simulink model "Der_Faux_FPGA_V2"  (R2020a)
settings: Solver=FixedStepDiscrete  StartTime=0.0  StopTime=0.84375  FixedStep=1/fs_sim  RelTol=1e-3
values from neighbouring files (symbols this model uses):
  ADC_res = 5    [Der_Faux_ctr_FPGA.m]
  ADC_res_G4 = 8    [Der_Faux_ctr_FPGA.m]
  C10 = 680e-12    (= 6.8e-10)    [Der_Faux_ctr_FPGA.m]
  C11 = 1e-9    (= 1e-09)    [Der_Faux_ctr_FPGA.m]
  C12 = 68e-9    (= 6.8e-08)    [Der_Faux_ctr_FPGA.m]
  C13 = 150e-9    (= 1.5e-07)    [Der_Faux_ctr_FPGA.m]
  C17 = 1e-6    (= 1e-06)    [Der_Faux_ctr_FPGA.m]
  C18 = 100e-9    (= 1e-07)    [Der_Faux_ctr_FPGA.m]
  C20 = 1e-6    (= 1e-06)    [Der_Faux_ctr_FPGA.m]
  C5 = 100e-12    (= 1e-10)    [Der_Faux_ctr_FPGA.m]
  C7 = 1e-6    (= 1e-06)    [Der_Faux_ctr_FPGA.m]
  D4_FL = D4_opt.FractionLength    [Der_Faux_ctr_FPGA.m]
  D4_opt = sfi(D4,len_D)    [Der_Faux_ctr_FPGA.m]
  D4_WL = D4_opt.WordLength    [Der_Faux_ctr_FPGA.m]
  D7_FL = D7_opt.FractionLength    [Der_Faux_ctr_FPGA.m]
  D7_opt = sfi(D7,len_D)    [Der_Faux_ctr_FPGA.m]
  D7_WL = D7_opt.WordLength    [Der_Faux_ctr_FPGA.m]
  D8_FL = D8_opt.FractionLength    [Der_Faux_ctr_FPGA.m]
  D8_opt = sfi(D8,len_D)    [Der_Faux_ctr_FPGA.m]
  D8_WL = D8_opt.WordLength    [Der_Faux_ctr_FPGA.m]
  Dcs1_FL = Dcs1_opt.FractionLength    [Der_Faux_ctr_FPGA.m]
  Dcs1_opt = sfi(Dcs1,len_D)    [Der_Faux_ctr_FPGA.m]
  Dcs1_WL = Dcs1_opt.WordLength    [Der_Faux_ctr_FPGA.m]
  Dcs2_FL = Dcs2_opt.FractionLength    [Der_Faux_ctr_FPGA.m]
  Dcs2_WL = Dcs2_opt.WordLength    [Der_Faux_ctr_FPGA.m]
  FP_frac = FP_len-10    (= 36)    [Der_Faux_ctr_FPGA.m]
  FP_len = 46    [Der_Faux_ctr_FPGA.m]
  fs = 48000    [Der_Faux_ctr_FPGA.m]
  fs_sim = fs*ovs    (= 6144000)    [Der_Faux_ctr_FPGA.m]
  G0 = 1/4.7e3    (= 0.000212765957447)    [Der_Faux_ctr_FPGA.m]
  G1 = 1/4.7e3    (= 0.000212765957447)    [Der_Faux_ctr_FPGA.m]
  G10 = 1/12e3    (= 8.33333333333e-05)    [Der_Faux_ctr_FPGA.m]
  G11 = 1/12e3    (= 8.33333333333e-05)    [Der_Faux_ctr_FPGA.m]
  G12 = 1/12e3    (= 8.33333333333e-05)    [Der_Faux_ctr_FPGA.m]
  G13 = 1/47e3    (= 2.12765957447e-05)    [Der_Faux_ctr_FPGA.m]
  G14 = 1/22e3    (= 4.54545454545e-05)    [Der_Faux_ctr_FPGA.m]
  G15 = 1/12e3    (= 8.33333333333e-05)    [Der_Faux_ctr_FPGA.m]
  G16 = 1/12e3    (= 8.33333333333e-05)    [Der_Faux_ctr_FPGA.m]
  G17 = 1/12e3    (= 8.33333333333e-05)    [Der_Faux_ctr_FPGA.m]
  G18 = 1/2.7e3    (= 0.00037037037037)    [Der_Faux_ctr_FPGA.m]
  G19 = 1/20e3    (= 5e-05)    [Der_Faux_ctr_FPGA.m]
  G20 = 1/10e3    (= 0.0001)    [Der_Faux_ctr_FPGA.m]
  G21 = 1/10e3    (= 0.0001)    [Der_Faux_ctr_FPGA.m]
  G5 = 1/22e3    (= 4.54545454545e-05)    [Der_Faux_ctr_FPGA.m]
  G7 = 1/12e3    (= 8.33333333333e-05)    [Der_Faux_ctr_FPGA.m]
  Gdem = 0.00096    [Der_Faux_ctr_FPGA.m]
  Gmod = 0.00096    [Der_Faux_ctr_FPGA.m]
  Gvar1_N = fi(Gvar1_N,0,ADC_res,0)    [Der_Faux_ctr_FPGA.m]
  Gvar2_N = fi(Gvar2_N,0,ADC_res,0)    [Der_Faux_ctr_FPGA.m]
  Gvar3_N = fi(Gvar3_N,0,ADC_res,0)    [Der_Faux_ctr_FPGA.m]
  Gvar4_N = fi(Gvar4_N,0,ADC_res_G4,0)    [Der_Faux_ctr_FPGA.m]
  input_space = linspace(0,2^ADC_res-1,2^ADC_res)    [Der_Faux_ctr_FPGA.m]
  input_space_G4 = linspace(0,2^ADC_res_G4-1,2^ADC_res_G4)    [Der_Faux_ctr_FPGA.m]
  input_spcae_extended = linspace(0,(2^ADC_res)^3-1,(2^ADC_res)^3)    [Der_Faux_ctr_FPGA.m]
  limit_Faux = 4.5    [Der_Faux_ctr_FPGA.m]
  limit_PT2399 = 2.5    [Der_Faux_ctr_FPGA.m]
  LUT_cd = fi(LUT_cd,0,LUT_cd_res,0)    [Der_Faux_ctr_FPGA.m]
  LUT_Gvar1_opt = sfi(LUT_Gvar1, len1)    [Der_Faux_ctr_FPGA.m]
  LUT_Gvar2_reversed_opt = sfi(LUT_Gvar2_reversed, len2)    [Der_Faux_ctr_FPGA.m]
  LUT_Gvar3_opt = sfi(LUT_Gvar3, len3)    [Der_Faux_ctr_FPGA.m]
  LUT_Z22a_opt = sfi(LUT_Z22a, len_LUT22a)    [Der_Faux_ctr_FPGA.m]
  LUT_Z22b_opt = sfi(LUT_Z22b, len_LUT22b)    [Der_Faux_ctr_FPGA.m]
  LUT_Z23a_opt = sfi(LUT_Z23a, len_Z23a)    [Der_Faux_ctr_FPGA.m]
  LUT_Z23b_opt = sfi(LUT_Z23b, len_Z23b)    [Der_Faux_ctr_FPGA.m]
  LUT_Z24a_opt = sfi(LUT_Z24a, len_LUT24a)    [Der_Faux_ctr_FPGA.m]
  LUT_Z24b_opt = sfi(LUT_Z24b, len_LUT24b)    [Der_Faux_ctr_FPGA.m]
  LUT_Z25a_opt = sfi(LUT_Z25a, len_LUT25a)    [Der_Faux_ctr_FPGA.m]
  LUT_Z25b_opt = sfi(LUT_Z25b, len_LUT25b)    [Der_Faux_ctr_FPGA.m]
  N4_FL = N4_opt.FractionLength    [Der_Faux_ctr_FPGA.m]
  N4_opt = sfi(N4,len_N)    [Der_Faux_ctr_FPGA.m]
  N4_WL = N4_opt.WordLength    [Der_Faux_ctr_FPGA.m]
  N7_FL = N7_opt.FractionLength    [Der_Faux_ctr_FPGA.m]
  N7_opt = sfi(N7,len_N)    [Der_Faux_ctr_FPGA.m]
  N7_WL = N7_opt.WordLength    [Der_Faux_ctr_FPGA.m]
  N8_FL = N8_opt.FractionLength    [Der_Faux_ctr_FPGA.m]
  N8_opt = sfi(N8,len_N)    [Der_Faux_ctr_FPGA.m]
  N8_WL = N8_opt.WordLength    [Der_Faux_ctr_FPGA.m]
  Ncs1_FL = Ncs1_opt.FractionLength    [Der_Faux_ctr_FPGA.m]
  Ncs1_opt = sfi(Ncs1,len_N)    [Der_Faux_ctr_FPGA.m]
  Ncs1_WL = Ncs1_opt.WordLength    [Der_Faux_ctr_FPGA.m]
  Ncs2_FL = Ncs2_opt.FractionLength    [Der_Faux_ctr_FPGA.m]
  Ncs2_WL = Ncs2_opt.WordLength    [Der_Faux_ctr_FPGA.m]
  shift_reg_size = 8*44000    (= 352000)    [Der_Faux_ctr_FPGA.m]
  use_stimuli = [true,true,true,true]    [Der_Faux_ctr_FPGA.m]
  w1 = 1e6    (= 1000000)    [Der_Faux_ctr_FPGA.m]
  w3 = 1e6    (= 1000000)    [Der_Faux_ctr_FPGA.m]
  w4 = 1e6    (= 1000000)    [Der_Faux_ctr_FPGA.m]
  w5 = 1e6    (= 1000000)    [Der_Faux_ctr_FPGA.m]
  w8 = 2*pi*3e6    (= 18849555.9215)    [Der_Faux_ctr_FPGA.m]
  WL_RAM = 5    [Der_Faux_ctr_FPGA.m]
undefined symbols (not defined in the file or in its folder): D10_FL, D10_opt, D10_WL, D11_FL, D11_opt, D11_WL, D13_FL, D13_opt, D13_WL, D16_FL, D16_opt, D16_WL, D20_FL, D20_opt, D20_WL, D21_FL, D21_opt, D21_WL, D26_FL, D26_opt, D26_WL, D27_FL, D27_opt, D27_WL, D28_FL, D28_opt, D28_WL, D29_FL, D29_opt, D29_WL, D30_FL, D30_opt, D30_WL, Dcs2, DiscIntNeverNeededParam, N10_FL, N10_opt, N10_WL, N11_FL, N11_opt, N11_WL, N13_FL, N13_opt, N13_WL, N16_FL, N16_opt, N16_WL, N20_FL, N20_opt, N20_WL, N21_FL, N21_opt, N21_WL, N26_FL, N26_opt, N26_WL, N27_FL, N27_opt, N27_WL, N28_FL ... (+13)
libraries: simulink x18, hdlsllib x4
(part 1 of 2)
settings Model: Creator=Donut  LastModifiedBy=Donut
settings OptimizationCC: BlockReduction=off  ConditionallyExecuteInputs=off  DefaultParameterBehavior=Inlined
settings DebuggingCC: SignalRangeChecking=warning  AlgebraicLoopMsg=error  SingleTaskRateTransMsg=error  ParameterOverflowMsg=warning  ParameterUnderflowMsg=warning  UnnecessaryDatatypeConvMsg=warning
settings HardwareCC: ProdBitPerPointer=32  ProdBitPerSizeT=32  ProdBitPerPtrDiffT=32  ProdLargestAtomicFloat=None  ProdIntDivRoundTo=Undefined  ProdEndianess=Unspecified  ProdWordSize=32  ProdHWDeviceType=ASIC/FPGA->ASIC/FPGA  TargetBitPerPointer=64  TargetBitPerSizeT=64  TargetBitPerPtrDiffT=64  TargetLongLongMode=on  TargetIntDivRoundTo=Zero  TargetEndianess=LittleEndian  TargetWordSize=64  TargetHWDeviceType=Custom Processor->MATLAB Host Computer  ProdEqTarget=off
settings SFSimCC: CustomCodeUndefinedFunction=UseInterfaceOnly

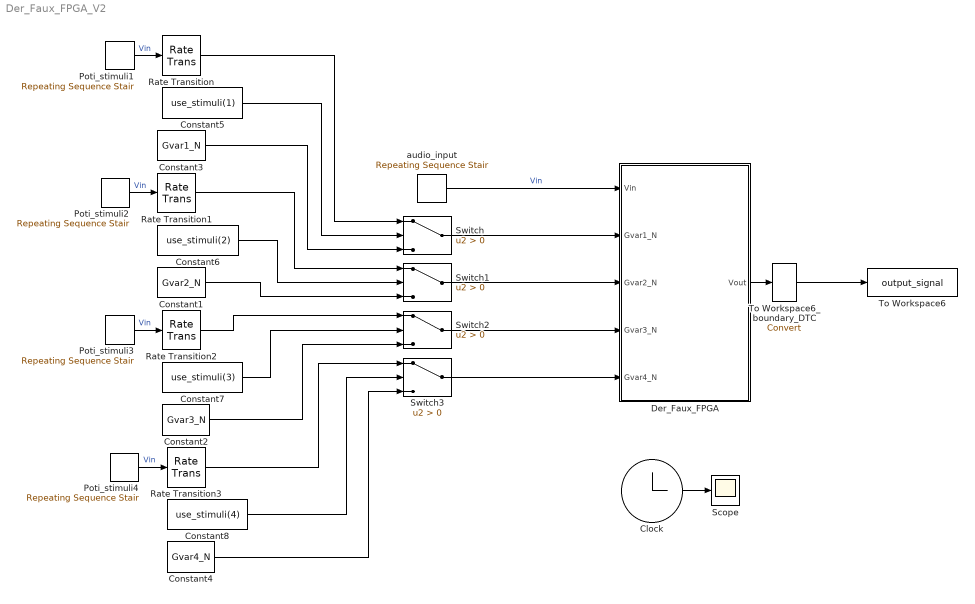
== system Der_Faux_FPGA_V2 ==
  Clock : Clock
  Constant1 : Constant  Value=Gvar2_N  OutDataTypeStr=fixdt(0,ADC_res,0)  SampleTime=1/fs_sim  LockScale=on
  Constant2 : Constant  Value=Gvar3_N  OutDataTypeStr=fixdt(0,ADC_res,0)  SampleTime=1/fs_sim  LockScale=on
  Constant3 : Constant  Value=Gvar1_N  OutDataTypeStr=fixdt(0,ADC_res,0)  SampleTime=1/fs_sim  LockScale=on
  Constant4 : Constant  Value=Gvar4_N  OutDataTypeStr=fixdt(0,ADC_res_G4,0)  SampleTime=1/(fs_sim)  LockScale=on
  Constant5 : Constant  Value=use_stimuli(1)  OutDataTypeStr=boolean  SampleTime=1/fs_sim  LockScale=on
  Constant6 : Constant  Value=use_stimuli(2)  OutDataTypeStr=boolean  SampleTime=1/fs_sim  LockScale=on
  Constant7 : Constant  Value=use_stimuli(3)  OutDataTypeStr=boolean  SampleTime=1/fs_sim  LockScale=on
  Constant8 : Constant  Value=use_stimuli(4)  OutDataTypeStr=boolean  SampleTime=1/(fs_sim)  LockScale=on
  Der_Faux_FPGA : Subsystem
  "Poti_stimuli1 " : simulink/Sources/Repeating Sequence Stair  OutValues=poti_stimuli1'  tsamp=1/fs  OutMin=[]  OutMax=[]  OutDataTypeStr=fixdt(0,ADC_res,0)  OutputDataTypeScalingMode=Specify via dialog  OutDataType=fixdt(0,ADC_res,0)  ConRadixGroup=Best Precision: Vector-wise  OutScaling=[]
      settings: LockScale=on
  "Poti_stimuli2 " : simulink/Sources/Repeating Sequence Stair  OutValues=poti_stimuli2'  tsamp=1/fs  OutMin=[]  OutMax=[]  OutDataTypeStr=fixdt(0,ADC_res,0)  OutputDataTypeScalingMode=Specify via dialog  OutDataType=fixdt(0,ADC_res,0)  ConRadixGroup=Best Precision: Vector-wise  OutScaling=[]
      settings: LockScale=on
  Poti_stimuli3 : simulink/Sources/Repeating Sequence Stair  OutValues=poti_stimuli3'  tsamp=1/fs  OutMin=[]  OutMax=[]  OutDataTypeStr=fixdt(0,ADC_res,0)  OutputDataTypeScalingMode=Specify via dialog  OutDataType=fixdt(0,ADC_res,0)  ConRadixGroup=Best Precision: Vector-wise  OutScaling=[]
      settings: LockScale=on
  Poti_stimuli4 : simulink/Sources/Repeating Sequence Stair  OutValues=poti_stimuli4'  tsamp=1/fs  OutMin=[]  OutMax=[]  OutDataTypeStr=fixdt(0,ADC_res_G4,0)  OutputDataTypeScalingMode=Specify via dialog  OutDataType=fixdt(0,ADC_res_G4,0)  ConRadixGroup=Best Precision: Vector-wise  OutScaling=[]
      settings: LockScale=on
  Rate Transition{,1..3} (4 alike) : RateTransition  OutPortSampleTime=1/fs_sim
  Scope : Scope
  Switch : Switch  Criteria=u2 > Threshold  OutDataTypeStr=fixdt(0,ADC_res,0)
      settings: LockScale=on
  Switch1 : Switch  Criteria=u2 > Threshold  OutDataTypeStr=fixdt(0,ADC_res,0)
      settings: LockScale=on
  Switch2 : Switch  Criteria=u2 > Threshold  OutDataTypeStr=fixdt(0,ADC_res,0)
      settings: LockScale=on
  Switch3 : Switch  Criteria=u2 > Threshold  OutDataTypeStr=fixdt(0,ADC_res_G4,0)
      settings: LockScale=on
  To Workspace6 : ToWorkspace  VariableName=output_signal  SaveFormat=Timeseries  SampleTime=1/fs
  To Workspace6_boundary_DTC : DataTypeConversion  SaturateOnIntegerOverflow=on  RndMeth=Zero
  audio_input : simulink/Sources/Repeating Sequence Stair  OutValues=audio'  tsamp=1/fs  OutMin=[]  OutMax=[]  OutDataTypeStr=fixdt(1,16,15)  OutputDataTypeScalingMode=Specify via dialog  OutDataType=fixdt(1,16,15)  ConRadixGroup=Best Precision: Vector-wise  OutScaling=[]
      settings: LockScale=on
  wires:
  Clock/1 -> Scope/1
  Constant5/1 -> Switch/2
  Constant6/1 -> Switch1/2
  Constant8/1 -> Switch3/2
  Constant7/1 -> Switch2/2
  Constant3/1 -> Switch/3
  Constant1/1 -> Switch1/3
  Constant2/1 -> Switch2/3
  Constant4/1 -> Switch3/3
  "Poti_stimuli1 "/1 -> Rate Transition/1  "Vin"
  Rate Transition/1 -> Switch/1
  Rate Transition3/1 -> Switch3/1
  "Poti_stimuli2 "/1 -> Rate Transition1/1  "Vin"
  Poti_stimuli3/1 -> Rate Transition2/1  "Vin"
  Poti_stimuli4/1 -> Rate Transition3/1  "Vin"
  Rate Transition1/1 -> Switch1/1
  Rate Transition2/1 -> Switch2/1
  Switch/1 -> Der_Faux_FPGA/2(Gvar1_N)
  Switch1/1 -> Der_Faux_FPGA/3(Gvar2_N)
  Switch3/1 -> Der_Faux_FPGA/5(Gvar4_N)
  audio_input/1 -> Der_Faux_FPGA/1(Vin)  "Vin"
  Switch2/1 -> Der_Faux_FPGA/4(Gvar3_N)
  Der_Faux_FPGA/1(Vout) -> To Workspace6_boundary_DTC/1
  To Workspace6_boundary_DTC/1 -> To Workspace6/1

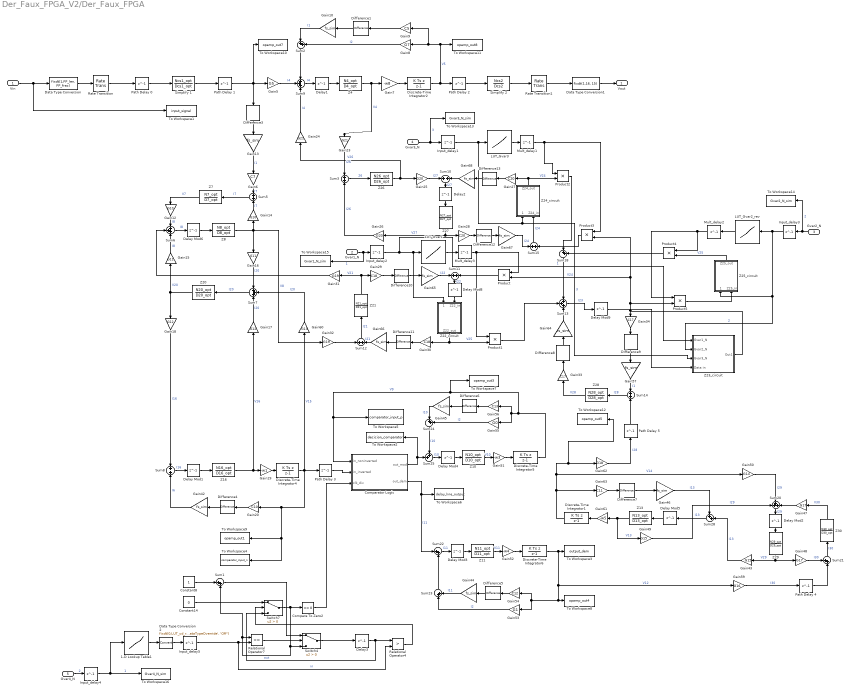
== system Der_Faux_FPGA_V2/Der_Faux_FPGA ==
  Vin : Inport  OutDataTypeStr=fixdt(1,16, 15)  SampleTime=1/fs  LockScale=on
  Gvar1_N : Inport  Port=2  OutDataTypeStr=fixdt(0,ADC_res,0, 'DataTypeOverride', 'Off')  SampleTime=1/fs_sim  LockScale=on
  Gvar2_N : Inport  Port=3  OutDataTypeStr=fixdt(0,ADC_res,0, 'DataTypeOverride', 'Off')  SampleTime=1/fs_sim  LockScale=on
  Gvar3_N : Inport  Port=4  OutDataTypeStr=fixdt(0,ADC_res,0, 'DataTypeOverride', 'Off')  SampleTime=1/fs_sim  LockScale=on
  Gvar4_N : Inport  Port=5  OutDataTypeStr=fixdt(0,ADC_res_G4,0, 'DataTypeOverride', 'Off')  SampleTime=1/(fs_sim)  LockScale=on
  1-D Lookup Table1 : Lookup_n-D  NumberOfTableDimensions=1  LookupTableObject=''  BreakpointsForDimension1=input_space_G4  BreakpointsForDimension1FirstPoint=10  BreakpointsForDimension2FirstPoint=10  BreakpointsForDimension1Spacing=12  BreakpointsForDimension2Spacing=12  BreakpointsForDimension1DataTypeStr=Inherit: Inherit from 'Breakpoint data'  IndexSearchMethod=Evenly spaced points  Table=LUT_cd  TableDataTypeStr=Inherit: Inherit from 'Table data'  InterpMethod=Flat  DiagnosticForOutOfRangeInput=Error  InternalRulePriority=Speed  OutDataTypeStr=Inherit: Inherit from 'Table data'  RndMeth=Simplest  InputSameDT=on  LockScale=on
  Comparator Logic : Subsystem
  Compare To Zero2 : simulink/Logic and Bit Operations/Compare To Zero  relop===  OutDataTypeStr=boolean
  Constant14 : Constant  Value=0  OutDataTypeStr=fixdt(0,LUT_cd_res,0, 'DataTypeOverride', 'Off')  SampleTime=1/(fs_sim)  LockScale=on
  Constant8 : Constant  OutDataTypeStr=fixdt(0,LUT_cd_res,0, 'DataTypeOverride', 'Off')  SampleTime=1/(fs_sim)  LockScale=on
  Data Type Conversion : DataTypeConversion  OutDataTypeStr=fixdt(1,FP_len, FP_frac)  SaturateOnIntegerOverflow=on
  Data Type Conversion1 : DataTypeConversion  OutDataTypeStr=fixdt(1,16, 15)  SaturateOnIntegerOverflow=on  LockScale=on
  Data Type Conversion2 : DataTypeConversion  OutDataTypeStr=fixdt(0,LUT_cd_res,0, 'DataTypeOverride', 'Off')  LockScale=on
  Delay Mod{1..6,8..9} (8 alike) : Delay  DelayLength=1  InitialCondition=0  SampleTime=1/fs_sim
  Delay1 : Delay  DelayLength=1
  Delay2 : Delay  DelayLength=1
  Delay3 : Delay  DelayLength=1  SampleTime=1/(fs_sim)
  Difference{1,3..13} (12 alike) : simulink/Discrete/Difference  ICPrevInput=0.0  OutMin=[]  OutMax=[]  OutDataTypeStr=fixdt(1,FP_len, FP_frac)  OutputDataTypeScalingMode=Specify via dialog  OutDataType=fixdt(1,FP_len, FP_frac)  OutScaling=[]  DoSatur=on
  Discrete-Time Integrator{1,4..6} (4 alike) : DiscreteIntegrator  IntegratorMethod=Integration: Backward Euler  SampleTime=1/fs_sim  OutDataTypeStr=fixdt(1,FP_len, FP_frac)  SaturateOnIntegerOverflow=on  LimitOutput=on  UpperSaturationLimit=limit_PT2399  LowerSaturationLimit=-limit_PT2399  ICPrevOutput=DiscIntNeverNeededParam  ICPrevScaledInput=DiscIntNeverNeededParam
  Discrete-Time Integrator2 : DiscreteIntegrator  IntegratorMethod=Integration: Backward Euler  SampleTime=1/fs_sim  OutDataTypeStr=fixdt(1,FP_len, FP_frac)  SaturateOnIntegerOverflow=on  LimitOutput=on  UpperSaturationLimit=limit_Faux  LowerSaturationLimit=-limit_Faux  ICPrevOutput=DiscIntNeverNeededParam  ICPrevScaledInput=DiscIntNeverNeededParam
  Gain{10,13,42,44..46,57,64..68} (12 alike) : Gain  Gain=fs_sim  OutDataTypeStr=fixdt(1,FP_len, FP_frac)  SaturateOnIntegerOverflow=on
  Gain12 : Gain  Gain=G10  OutDataTypeStr=fixdt(1,FP_len, FP_frac)  SaturateOnIntegerOverflow=on
  Gain14 : Gain  Gain=G10  OutDataTypeStr=fixdt(1,FP_len, FP_frac)  SaturateOnIntegerOverflow=on
  Gain15 : Gain  Gain=G11  OutDataTypeStr=fixdt(1,FP_len, FP_frac)  SaturateOnIntegerOverflow=on
  Gain16 : Gain  Gain=G11  OutDataTypeStr=fixdt(1,FP_len, FP_frac)  SaturateOnIntegerOverflow=on
  Gain17 : Gain  Gain=G12  OutDataTypeStr=fixdt(1,FP_len, FP_frac)  SaturateOnIntegerOverflow=on
  Gain18 : Gain  Gain=G12  OutDataTypeStr=fixdt(1,FP_len, FP_frac)  SaturateOnIntegerOverflow=on
  Gain19 : Gain  Gain=-w1  OutDataTypeStr=fixdt(1,FP_len, FP_frac)  SaturateOnIntegerOverflow=on
  Gain20 : Gain  Gain=C10  OutDataTypeStr=fixdt(1,FP_len, FP_frac)  SaturateOnIntegerOverflow=on
  Gain23 : Gain  Gain=G21  OutDataTypeStr=fixdt(1,FP_len, FP_frac)  SaturateOnIntegerOverflow=on
  Gain24 : Gain  Gain=G21  OutDataTypeStr=fixdt(1,FP_len, FP_frac)  SaturateOnIntegerOverflow=on
  Gain25 : Gain  Gain=G20  OutDataTypeStr=fixdt(1,FP_len, FP_frac)  SaturateOnIntegerOverflow=on
  Gain26 : Gain  Gain=G20  OutDataTypeStr=fixdt(1,FP_len, FP_frac)  SaturateOnIntegerOverflow=on
  Gain27 : Gain  Gain=C20  OutDataTypeStr=fixdt(1,FP_len, FP_frac)  SaturateOnIntegerOverflow=on
  Gain28 : Gain  Gain=C20  OutDataTypeStr=fixdt(1,FP_len, FP_frac)  SaturateOnIntegerOverflow=on
  Gain29 : Gain  Gain=C18  OutDataTypeStr=fixdt(1,FP_len, FP_frac)  SaturateOnIntegerOverflow=on
  Gain30 : Gain  Gain=C18  OutDataTypeStr=fixdt(1,FP_len, FP_frac)  SaturateOnIntegerOverflow=on
  Gain31 : Gain  Gain=G19  OutDataTypeStr=fixdt(1,FP_len, FP_frac)  SaturateOnIntegerOverflow=on
  Gain32 : Gain  Gain=G19  OutDataTypeStr=fixdt(1,FP_len, FP_frac)  SaturateOnIntegerOverflow=on
  Gain33 : Gain  Gain=C17  OutDataTypeStr=fixdt(1,FP_len, FP_frac)  SaturateOnIntegerOverflow=on
  Gain34 : Gain  Gain=C17  OutDataTypeStr=fixdt(1,FP_len, FP_frac)  SaturateOnIntegerOverflow=on
  Gain43 : Gain  Gain=G15  OutDataTypeStr=fixdt(1,FP_len, FP_frac)  SaturateOnIntegerOverflow=on
  Gain47 : Gain  Gain=G17  OutDataTypeStr=fixdt(1,FP_len, FP_frac)  SaturateOnIntegerOverflow=on
  Gain48 : Gain  Gain=G17  OutDataTypeStr=fixdt(1,FP_len, FP_frac)  SaturateOnIntegerOverflow=on
  Gain49 : Gain  Gain=G15  OutDataTypeStr=fixdt(1,FP_len, FP_frac)  SaturateOnIntegerOverflow=on
  Gain5 : Gain  Gain=G5  OutDataTypeStr=fixdt(1,FP_len, FP_frac)  SaturateOnIntegerOverflow=on
  Gain50 : Gain  Gain=G14  OutDataTypeStr=fixdt(1,FP_len, FP_frac)  SaturateOnIntegerOverflow=on
  Gain51 : Gain  Gain=-w3  OutDataTypeStr=fixdt(1,FP_len, FP_frac)  SaturateOnIntegerOverflow=on
  Gain52 : Gain  Gain=-w4  OutDataTypeStr=fixdt(1,FP_len, FP_frac)  SaturateOnIntegerOverflow=on
  Gain53 : Gain  Gain=G1  OutDataTypeStr=fixdt(1,FP_len, FP_frac)  SaturateOnIntegerOverflow=on
  Gain54 : Gain  Gain=C12  OutDataTypeStr=fixdt(1,FP_len, FP_frac)  SaturateOnIntegerOverflow=on
  Gain55 : Gain  Gain=G0  OutDataTypeStr=fixdt(1,FP_len, FP_frac)  SaturateOnIntegerOverflow=on
  Gain56 : Gain  Gain=C13  OutDataTypeStr=fixdt(1,FP_len, FP_frac)  SaturateOnIntegerOverflow=on
  Gain59 : Gain  Gain=G16  OutDataTypeStr=fixdt(1,FP_len, FP_frac)  SaturateOnIntegerOverflow=on
  Gain6 : Gain  Gain=C7  OutDataTypeStr=fixdt(1,FP_len, FP_frac)  SaturateOnIntegerOverflow=on
  Gain60 : Gain  Gain=G13  OutDataTypeStr=fixdt(1,FP_len, FP_frac)  SaturateOnIntegerOverflow=on
  Gain61 : Gain  Gain=-w5  OutDataTypeStr=fixdt(1,FP_len, FP_frac)  SaturateOnIntegerOverflow=on
  Gain62 : Gain  Gain=G18  OutDataTypeStr=fixdt(1,FP_len, FP_frac)  SaturateOnIntegerOverflow=on
  Gain63 : Gain  Gain=C11  OutDataTypeStr=fixdt(1,FP_len, FP_frac)  SaturateOnIntegerOverflow=on
  Gain7 : Gain  Gain=-w8  OutDataTypeStr=fixdt(1,FP_len, FP_frac)  SaturateOnIntegerOverflow=on
  Gain8 : Gain  Gain=G7  OutDataTypeStr=fixdt(1,FP_len, FP_frac)  SaturateOnIntegerOverflow=on
  Gain9 : Gain  Gain=C5  OutDataTypeStr=fixdt(1,FP_len, FP_frac)  SaturateOnIntegerOverflow=on
  Input_delay{1..4} (4 alike) : Delay  DelayLength=1
  Input_delay5 : Delay  DelayLength=1  InitialCondition=1  SampleTime=1/(fs_sim)
  "LUT_Gvar1 " : Lookup_n-D  NumberOfTableDimensions=1  LookupTableObject=''  BreakpointsForDimension1=input_space  BreakpointsForDimension1FirstPoint=10  BreakpointsForDimension2FirstPoint=10  BreakpointsForDimension1Spacing=12  BreakpointsForDimension2Spacing=12  IndexSearchMethod=Evenly spaced points  Table=LUT_Gvar1_opt  TableDataTypeStr=Inherit: Inherit from 'Table data'  InterpMethod=Flat  DiagnosticForOutOfRangeInput=Error  InternalRulePriority=Speed  OutDataTypeStr=Inherit: Inherit from 'Table data'  RndMeth=Simplest  InputSameDT=on  LockScale=on
  LUT_Gvar2_rev : Lookup_n-D  NumberOfTableDimensions=1  LookupTableObject=''  BreakpointsForDimension1=input_space  BreakpointsForDimension1FirstPoint=10  BreakpointsForDimension2FirstPoint=10  BreakpointsForDimension1Spacing=12  BreakpointsForDimension2Spacing=12  BreakpointsForDimension1DataTypeStr=Inherit: Inherit from 'Breakpoint data'  IndexSearchMethod=Evenly spaced points  Table=LUT_Gvar2_reversed_opt  TableDataTypeStr=Inherit: Inherit from 'Table data'  InterpMethod=Flat  DiagnosticForOutOfRangeInput=Error  InternalRulePriority=Speed  OutDataTypeStr=Inherit: Inherit from 'Table data'  RndMeth=Simplest  InputSameDT=on  LockScale=on
  "LUT_Gvar3 " : Lookup_n-D  NumberOfTableDimensions=1  LookupTableObject=''  BreakpointsForDimension1=input_space  BreakpointsForDimension1FirstPoint=10  BreakpointsForDimension2FirstPoint=10  BreakpointsForDimension1Spacing=12  BreakpointsForDimension2Spacing=12  BreakpointsForDimension1DataTypeStr=Inherit: Inherit from 'Breakpoint data'  IndexSearchMethod=Evenly spaced points  Table=LUT_Gvar3_opt  TableDataTypeStr=Inherit: Inherit from 'Table data'  InterpMethod=Flat  DiagnosticForOutOfRangeInput=Error  InternalRulePriority=Speed  OutDataTypeStr=Inherit: Inherit from 'Table data'  RndMeth=Simplest  InputSameDT=on  LockScale=on
  Mult_delay1 : Delay  DelayLength=1
  Mult_delay2 : Delay  DelayLength=1
  Mult_delay3 : Delay  DelayLength=1
  Path Delay {0..5} (6 alike) : Delay  DelayLength=1
  Product{,1..5} (6 alike) : Product  OutDataTypeStr=fixdt(1,FP_len, FP_frac)  SaturateOnIntegerOverflow=on
  Rate Transition : RateTransition  OutPortSampleTime=1/fs_sim
  Rate Transition1 : RateTransition  OutPortSampleTimeOpt=Multiple of input port sample time  OutPortSampleTimeMultiple=ovs  OutPortSampleTime=1/fs
  Relational Operator4 : RelationalOperator  Operator=>  OutDataTypeStr=boolean  RndMeth=Nearest
  Relational Operator7 : RelationalOperator  Operator=<=  OutDataTypeStr=boolean  RndMeth=Nearest
  Simplify 1 : DiscreteTransferFcn  Numerator=Ncs1_opt  Denominator=Dcs1_opt  SampleTime=1/fs_sim  StateDataTypeStr=fixdt(1,FP_len, FP_frac)  NumCoefDataTypeStr=fixdt(1,Ncs1_WL, Ncs1_FL)  DenCoefDataTypeStr=fixdt(1,Dcs1_WL, Dcs1_FL)  NumProductDataTypeStr=fixdt(1,FP_len, FP_frac)  DenProductDataTypeStr=fixdt(1,FP_len, FP_frac)  NumAccumDataTypeStr=fixdt(1,FP_len, FP_frac)  DenAccumDataTypeStr=fixdt(1,FP_len, FP_frac)  OutDataTypeStr=fixdt(1,FP_len, FP_frac)  SaturateOnIntegerOverflow=on
  Simplify 2 : DiscreteTransferFcn  Numerator=Ncs2  Denominator=Dcs2  SampleTime=1/fs_sim  a0EqualsOne=on  StateDataTypeStr=fixdt(1,FP_len, FP_frac)  NumCoefDataTypeStr=fixdt(1,Ncs2_WL, Ncs2_FL)  DenCoefDataTypeStr=fixdt(1,Dcs2_WL, Dcs2_FL)  NumProductDataTypeStr=fixdt(1,FP_len, FP_frac)  DenProductDataTypeStr=fixdt(1,FP_len, FP_frac)  NumAccumDataTypeStr=fixdt(1,FP_len, FP_frac)  DenAccumDataTypeStr=fixdt(1,FP_len, FP_frac)  OutDataTypeStr=fixdt(1,FP_len, FP_frac)  SaturateOnIntegerOverflow=on
  Sum1 : Sum  Inputs=|++  OutDataTypeStr=fixdt(0,LUT_cd_res,0, 'DataTypeOverride', 'Off')  LockScale=on
  Sum{3,5,8,10..12,14..15} (8 alike) : Sum  Inputs=+|+  OutDataTypeStr=fixdt(1,FP_len, FP_frac)  SaturateOnIntegerOverflow=on
  Sum{6..7,9,13,20} (5 alike) : Sum  Inputs=+++  OutDataTypeStr=fixdt(1,FP_len, FP_frac)  SaturateOnIntegerOverflow=on
  Sum{2,18,22..24} (5 alike) : Sum  Inputs=|++  OutDataTypeStr=fixdt(1,FP_len, FP_frac)  SaturateOnIntegerOverflow=on
  Sum21 : Sum  Inputs=++|  OutDataTypeStr=fixdt(1,FP_len, FP_frac)  SaturateOnIntegerOverflow=on
  Sum25 : Sum  Inputs=++|  OutDataTypeStr=fixdt(1,FP_len, FP_frac)  SaturateOnIntegerOverflow=on
  Sum28 : Sum  Inputs=++|  OutDataTypeStr=fixdt(1,FP_len, FP_frac)  SaturateOnIntegerOverflow=on
  Switch4 : Switch  Criteria=u2 > Threshold  OutDataTypeStr=fixdt(0,LUT_cd_res,0, 'DataTypeOverride', 'Off')
      settings: LockScale=on
  Switch7 : Switch  Criteria=u2 > Threshold  OutDataTypeStr=fixdt(0,LUT_cd_res,0, 'DataTypeOverride', 'Off')
      settings: LockScale=on
  To Workspace1 : ToWorkspace  VariableName=input_signal  SaveFormat=Timeseries  SampleTime=1/fs
  To Workspace10 : ToWorkspace  VariableName=opamp_out7  SaveFormat=Timeseries  SampleTime=-1
  To Workspace11 : ToWorkspace  VariableName=opamp_out8  SaveFormat=Timeseries  SampleTime=-1
  To Workspace12 : ToWorkspace  VariableName=opamp_out5  SaveFormat=Timeseries  SampleTime=-1
  To Workspace13 : ToWorkspace  VariableName=Gvar3_N_sim  SaveFormat=Timeseries  SampleTime=1/fs_sim
  To Workspace14 : ToWorkspace  VariableName=Gvar2_N_sim  SaveFormat=Timeseries  SampleTime=1/fs_sim
  To Workspace15 : ToWorkspace  VariableName=Gvar1_N_sim  SaveFormat=Timeseries  SampleTime=1/fs_sim
  To Workspace16 : ToWorkspace  VariableName=Gvar4_N_sim  SaveFormat=Timeseries  SampleTime=1/(fs_sim)
  To Workspace2 : ToWorkspace  VariableName=decicion_comparator  SaveFormat=Timeseries  SampleTime=-1
  To Workspace3 : ToWorkspace  VariableName=output_dem  SaveFormat=Timeseries  SampleTime=-1
  To Workspace4 : ToWorkspace  VariableName=comparator_input_n  SaveFormat=Timeseries  SampleTime=-1
  To Workspace5 : ToWorkspace  VariableName=comparator_input_p  SaveFormat=Timeseries  SampleTime=-1
  To Workspace6 : ToWorkspace  VariableName=delay_line_output  SaveFormat=Timeseries  SampleTime=-1
  To Workspace7 : ToWorkspace  VariableName=opamp_out3  SaveFormat=Timeseries  SampleTime=-1
  To Workspace8 : ToWorkspace  VariableName=opamp_out4  SaveFormat=Timeseries  SampleTime=-1
  To Workspace9 : ToWorkspace  VariableName=opamp_out1  SaveFormat=Timeseries  SampleTime=-1
  Z10 : DiscreteTransferFcn  Numerator=N10_opt  Denominator=D10_opt  SampleTime=1/fs_sim  StateDataTypeStr=fixdt(1,FP_len, FP_frac)  NumCoefDataTypeStr=fixdt(1,N10_WL, N10_FL)  DenCoefDataTypeStr=fixdt(1,D10_WL, D10_FL)  NumProductDataTypeStr=fixdt(1,FP_len, FP_frac)  DenProductDataTypeStr=fixdt(1,FP_len, FP_frac)  NumAccumDataTypeStr=fixdt(1,FP_len, FP_frac)  DenAccumDataTypeStr=fixdt(1,FP_len, FP_frac)  OutDataTypeStr=fixdt(1,FP_len, FP_frac)  SaturateOnIntegerOverflow=on
  Z11 : DiscreteTransferFcn  Numerator=N11_opt  Denominator=D11_opt  SampleTime=1/fs_sim  StateDataTypeStr=fixdt(1,FP_len, FP_frac)  NumCoefDataTypeStr=fixdt(1,N11_WL, N11_FL)  DenCoefDataTypeStr=fixdt(1,D11_WL, D11_FL)  NumProductDataTypeStr=fixdt(1,FP_len, FP_frac)  DenProductDataTypeStr=fixdt(1,FP_len, FP_frac)  NumAccumDataTypeStr=fixdt(1,FP_len, FP_frac)  DenAccumDataTypeStr=fixdt(1,FP_len, FP_frac)  OutDataTypeStr=fixdt(1,FP_len, FP_frac)  SaturateOnIntegerOverflow=on
  Z13 : DiscreteTransferFcn  Numerator=N13_opt  Denominator=D13_opt  SampleTime=1/fs_sim  StateDataTypeStr=fixdt(1,FP_len, FP_frac)  NumCoefDataTypeStr=fixdt(1,N13_WL, N13_FL)  DenCoefDataTypeStr=fixdt(1,D13_WL, D13_FL)  NumProductDataTypeStr=fixdt(1,FP_len, FP_frac)  DenProductDataTypeStr=fixdt(1,FP_len, FP_frac)  NumAccumDataTypeStr=fixdt(1,FP_len, FP_frac)  DenAccumDataTypeStr=fixdt(1,FP_len, FP_frac)  OutDataTypeStr=fixdt(1,FP_len, FP_frac)  SaturateOnIntegerOverflow=on
  Z16 : DiscreteTransferFcn  Numerator=N16_opt  Denominator=D16_opt  SampleTime=1/fs_sim  StateDataTypeStr=fixdt(1,FP_len, FP_frac)  NumCoefDataTypeStr=fixdt(1,N16_WL, N16_FL)  DenCoefDataTypeStr=fixdt(1,D16_WL, D16_FL)  NumProductDataTypeStr=fixdt(1,FP_len, FP_frac)  DenProductDataTypeStr=fixdt(1,FP_len, FP_frac)  NumAccumDataTypeStr=fixdt(1,FP_len, FP_frac)  DenAccumDataTypeStr=fixdt(1,FP_len, FP_frac)  OutDataTypeStr=fixdt(1,FP_len, FP_frac)  SaturateOnIntegerOverflow=on
  Z20 : DiscreteTransferFcn  Numerator=N20_opt  Denominator=D20_opt  SampleTime=1/fs_sim  StateDataTypeStr=fixdt(1,FP_len, FP_frac)  NumCoefDataTypeStr=fixdt(1,N20_WL, N20_FL)  DenCoefDataTypeStr=fixdt(1,D20_WL, D20_FL)  NumProductDataTypeStr=fixdt(1,FP_len, FP_frac)  DenProductDataTypeStr=fixdt(1,FP_len, FP_frac)  NumAccumDataTypeStr=fixdt(1,FP_len, FP_frac)  DenAccumDataTypeStr=fixdt(1,FP_len, FP_frac)  OutDataTypeStr=fixdt(1,FP_len, FP_frac)  SaturateOnIntegerOverflow=on
  Z21 : DiscreteTransferFcn  Numerator=N21_opt  Denominator=D21_opt  SampleTime=1/fs_sim  StateDataTypeStr=fixdt(1,FP_len, FP_frac)  NumCoefDataTypeStr=fixdt(1,N21_WL, N21_FL)  DenCoefDataTypeStr=fixdt(1,D21_WL, D21_FL)  NumProductDataTypeStr=fixdt(1,FP_len, FP_frac)  DenProductDataTypeStr=fixdt(1,FP_len, FP_frac)  NumAccumDataTypeStr=fixdt(1,FP_len, FP_frac)  DenAccumDataTypeStr=fixdt(1,FP_len, FP_frac)  OutDataTypeStr=fixdt(1,FP_len, FP_frac)  SaturateOnIntegerOverflow=on
  Z22_circuit : Subsystem
  Z23_circuit : Subsystem
  Z24_circuit : Subsystem
  Z25_circuit : Subsystem
  Z26 : DiscreteTransferFcn  Numerator=N26_opt  Denominator=D26_opt  SampleTime=1/fs_sim  StateDataTypeStr=fixdt(1,FP_len, FP_frac)  NumCoefDataTypeStr=fixdt(1,N26_WL, N26_FL)  DenCoefDataTypeStr=fixdt(1,D26_WL, D26_FL)  NumProductDataTypeStr=fixdt(1,FP_len, FP_frac)  DenProductDataTypeStr=fixdt(1,FP_len, FP_frac)  NumAccumDataTypeStr=fixdt(1,FP_len, FP_frac)  DenAccumDataTypeStr=fixdt(1,FP_len, FP_frac)  OutDataTypeStr=fixdt(1,FP_len, FP_frac)  SaturateOnIntegerOverflow=on
  Z27 : DiscreteTransferFcn  Numerator=N27_opt  Denominator=D27_opt  SampleTime=1/fs_sim  StateDataTypeStr=fixdt(1,FP_len, FP_frac)  NumCoefDataTypeStr=fixdt(1,N27_WL, N27_FL)  DenCoefDataTypeStr=fixdt(1,D27_WL, D27_FL)  NumProductDataTypeStr=fixdt(1,FP_len, FP_frac)  DenProductDataTypeStr=fixdt(1,FP_len, FP_frac)  NumAccumDataTypeStr=fixdt(1,FP_len, FP_frac)  DenAccumDataTypeStr=fixdt(1,FP_len, FP_frac)  OutDataTypeStr=fixdt(1,FP_len, FP_frac)  SaturateOnIntegerOverflow=on
  Z28 : DiscreteTransferFcn  Numerator=N28_opt  Denominator=D28_opt  SampleTime=1/fs_sim  StateDataTypeStr=fixdt(1,FP_len, FP_frac)  NumCoefDataTypeStr=fixdt(1,N28_WL, N28_FL)  DenCoefDataTypeStr=fixdt(1,D28_WL, D28_FL)  NumProductDataTypeStr=fixdt(1,FP_len, FP_frac)  DenProductDataTypeStr=fixdt(1,FP_len, FP_frac)  NumAccumDataTypeStr=fixdt(1,FP_len, FP_frac)  DenAccumDataTypeStr=fixdt(1,FP_len, FP_frac)  OutDataTypeStr=fixdt(1,FP_len, FP_frac)  SaturateOnIntegerOverflow=on
  Z29 : DiscreteTransferFcn  Numerator=N29_opt  Denominator=D29_opt  SampleTime=1/fs_sim  StateDataTypeStr=fixdt(1,FP_len, FP_frac)  NumCoefDataTypeStr=fixdt(1,N29_WL, N29_FL)  DenCoefDataTypeStr=fixdt(1,D29_WL, D29_FL)  NumProductDataTypeStr=fixdt(1,FP_len, FP_frac)  DenProductDataTypeStr=fixdt(1,FP_len, FP_frac)  NumAccumDataTypeStr=fixdt(1,FP_len, FP_frac)  DenAccumDataTypeStr=fixdt(1,FP_len, FP_frac)  OutDataTypeStr=fixdt(1,FP_len, FP_frac)  SaturateOnIntegerOverflow=on
  Z30 : DiscreteTransferFcn  Numerator=N30_opt  Denominator=D30_opt  SampleTime=1/fs_sim  StateDataTypeStr=fixdt(1,FP_len, FP_frac)  NumCoefDataTypeStr=fixdt(1,N30_WL, N30_FL)  DenCoefDataTypeStr=fixdt(1,D30_WL, D30_FL)  NumProductDataTypeStr=fixdt(1,FP_len, FP_frac)  DenProductDataTypeStr=fixdt(1,FP_len, FP_frac)  NumAccumDataTypeStr=fixdt(1,FP_len, FP_frac)  DenAccumDataTypeStr=fixdt(1,FP_len, FP_frac)  OutDataTypeStr=fixdt(1,FP_len, FP_frac)  SaturateOnIntegerOverflow=on
  "Z4 " : DiscreteTransferFcn  Numerator=N4_opt  Denominator=D4_opt  SampleTime=1/fs_sim  StateDataTypeStr=fixdt(1,FP_len, FP_frac)  NumCoefDataTypeStr=fixdt(1,N4_WL, N4_FL)  DenCoefDataTypeStr=fixdt(1,D4_WL, D4_FL)  NumProductDataTypeStr=fixdt(1,FP_len, FP_frac)  DenProductDataTypeStr=fixdt(1,FP_len, FP_frac)  NumAccumDataTypeStr=fixdt(1,FP_len, FP_frac)  DenAccumDataTypeStr=fixdt(1,FP_len, FP_frac)  OutDataTypeStr=fixdt(1,FP_len, FP_frac)  SaturateOnIntegerOverflow=on
  Z7 : DiscreteTransferFcn  Numerator=N7_opt  Denominator=D7_opt  SampleTime=1/fs_sim  StateDataTypeStr=fixdt(1,FP_len, FP_frac)  NumCoefDataTypeStr=fixdt(1,N7_WL, N7_FL)  DenCoefDataTypeStr=fixdt(1,D7_WL, D7_FL)  NumProductDataTypeStr=fixdt(1,FP_len, FP_frac)  DenProductDataTypeStr=fixdt(1,FP_len, FP_frac)  NumAccumDataTypeStr=fixdt(1,FP_len, FP_frac)  DenAccumDataTypeStr=fixdt(1,FP_len, FP_frac)  OutDataTypeStr=fixdt(1,FP_len, FP_frac)  SaturateOnIntegerOverflow=on
  Z8 : DiscreteTransferFcn  Numerator=N8_opt  Denominator=D8_opt  SampleTime=1/fs_sim  StateDataTypeStr=fixdt(1,FP_len, FP_frac)  NumCoefDataTypeStr=fixdt(1,N8_WL, N8_FL)  DenCoefDataTypeStr=fixdt(1,D8_WL, D8_FL)  NumProductDataTypeStr=fixdt(1,FP_len, FP_frac)  DenProductDataTypeStr=fixdt(1,FP_len, FP_frac)  NumAccumDataTypeStr=fixdt(1,FP_len, FP_frac)  DenAccumDataTypeStr=fixdt(1,FP_len, FP_frac)  OutDataTypeStr=fixdt(1,FP_len, FP_frac)  SaturateOnIntegerOverflow=on
  Vout : Outport
  wires:
  Sum3/1 -> Z26/1  "26"
  Difference13/1 -> Gain68/1
  Delay Mod2/1 -> Z29/1
  Gain10/1 -> Sum2/1  "I1"
  Gain34/1 -> Difference9/1
  Z27/1 -> Gain26/1, Gain28/1  "V27"
  Simplify 2/1 -> Rate Transition1/1
  Difference12/1 -> Gain67/1
  Sum11/1 -> Delay Mod8/1  "I22"
  Gain57/1 -> Sum14/1  "I1"
  Discrete-Time Integrator6/1 -> Gain53/1, Gain54/1, To Workspace8/1, Gain59/1, To Workspace3/1  "V12"
  Sum25/1 -> Delay Mod4/1  "I10"
  Discrete-Time Integrator2/1 -> Gain9/1, Gain8/1, To Workspace11/1, Path Delay 2/1  "V5"
  "Z4 "/1 -> Gain23/1, Gain7/1  "V4"
  Difference11/1 -> Gain66/1
  Gain67/1 -> Sum15/1  "I24"
  Delay Mod1/1 -> Z16/1
  Gain65/1 -> Sum11/1  "I22"
  Sum21/1 -> Z30/1  "I30"
  Gain50/1 -> Sum20/2  "I29"
  Sum13/1 -> Delay Mod9/1  "I23"
  Sum9/1 -> Delay1/1  "I4"
  Z29/1 -> Gain48/1, Gain43/1  "V29"
  Difference5/1 -> Gain44/1
  Sum22/1 -> Delay Mod3/1  "I11"
  Gain17/1 -> Sum7/3  "I20"
  Sum14/1 -> Z28/1  "I28"
  Delay Mod3/1 -> Z11/1
  Gain46/1 -> Sum28/1  "I13"
  Discrete-Time Integrator4/1 -> To Workspace4/1, To Workspace9/1, Gain20/1, Path Delay 3/1, Gain60/1  "V15"
  Z20/1 -> Gain15/1, Gain18/1  "V20"
  Sum28/1 -> Delay Mod5/1  "I13"
  Difference7/1 -> Gain46/1
  Gain31/1 -> Sum6/2
  Gain27/1 -> Difference13/1
  Discrete-Time Integrator1/1 -> Gain63/1, Gain50/1, Gain62/1, To Workspace12/1  "V14"
  Difference8/1 -> Gain64/1
  Gain14/1 -> Sum5/2  "I7"
  Gain5/1 -> Sum9/2  "I4"
  Difference9/1 -> Gain57/1
  Gain7/1 -> Discrete-Time Integrator2/1
  Delay Mod4/1 -> Z10/1
  Delay Mod5/1 -> Z13/1
  Gain30/1 -> Difference11/1
  Difference6/1 -> Gain45/1
  Sum20/1 -> Delay Mod2/1  "I29"
  Delay1/1 -> "Z4 "/1
  Sum6/1 -> Delay Mod6/1  "I8"
  Difference4/1 -> Gain42/1
  Gain56/1 -> Difference6/1
  Gain63/1 -> Difference7/1
  Gain32/1 -> Sum12/1
  Z10/1 -> Gain51/1  "V10"
  Gain45/1 -> Sum24/1  "I10"
  Gain43/1 -> Sum28/2  "I13"
  Gain12/1 -> Sum6/1  "I8"
  Difference10/1 -> Gain65/1
  Gain47/1 -> Sum20/3
  Sum8/1 -> Delay Mod1/1  "I16"
  Gain66/1 -> Sum12/2  "I21"
  Gain54/1 -> Difference5/1
  Z8/1 -> Gain32/1, Gain16/1, Gain14/1  "V8"
  Gain6/1 -> Sum5/1  "I7"
  Sum5/1 -> Z7/1  "I7"
  Gain16/1 -> Sum7/1  "I20"
  Z7/1 -> Gain12/1  "V7"
  Z21/1 -> Gain29/1, Gain31/1  "V21"
  Gain18/1 -> Sum8/1  "I16"
  Gain68/1 -> Sum10/2
  Sum2/1 -> Sum9/1
  Gain44/1 -> Sum23/2  "I11"
  Gain25/1 -> Sum10/1  "I27"
  Gain49/1 -> Sum20/1  "I29"
  Discrete-Time Integrator5/1 -> To Workspace7/1, Comparator Logic/1(in_noninverted), To Workspace5/1, Gain55/1, Gain56/1  "V9"
  Sum18/1 -> Sum13/1
  Comparator Logic/2(out_dem) -> To Workspace6/1, Sum22/1  "I11"
  Z11/1 -> Gain52/1  "V11"
  Sum23/1 -> Sum22/2
  Gain48/1 -> Sum21/1  "I30"
  Z30/1 -> Gain47/1  "V30"
  Gain55/1 -> Sum24/2  "I2"
  Gain8/1 -> Sum2/2  "I2"
  Z28/1 -> Gain33/1  "V28"
  Gain28/1 -> Difference12/1
  Gain51/1 -> Discrete-Time Integrator5/1
  Z13/1 -> Gain49/1, Gain61/1  "V13"
  Gain19/1 -> Discrete-Time Integrator4/1
  Gain64/1 -> Sum13/3
  Gain59/1 -> Path Delay 4/1  "I30"
  Gain60/1 -> Sum7/2  "I20"
  Gain52/1 -> Discrete-Time Integrator6/1
  Z26/1 -> Gain24/1, Gain25/1  "V26"
  Gain53/1 -> Sum23/1  "I2"
  Sum24/1 -> Sum25/1  "I10"
  Rate Transition/1 -> Path Delay 0/1
  Gain15/1 -> Sum6/3  "I8"
  Gain26/1 -> Sum3/2  "I26"
  Gain61/1 -> Discrete-Time Integrator1/1
  Sum12/1 -> Z21/1  "I21"
  Z16/1 -> Gain19/1, Gain17/1  "V16"
  Gain23/1 -> Sum3/1  "I26"
  Difference1/1 -> Gain10/1
  Difference3/1 -> Gain13/1
  Gain9/1 -> Difference1/1
  Gain29/1 -> Difference10/1
  Gain13/1 -> Gain6/1  "I1"
  Gain20/1 -> Difference4/1
  Gain33/1 -> Difference8/1
  Sum7/1 -> Z20/1  "I20"
  Gain42/1 -> Sum8/2  "I6"
  Comparator Logic/1(out_mod) -> To Workspace2/1, Sum25/2
  Simplify 1/1 -> Path Delay 1/1
  Gain62/1 -> Path Delay 5/1  "I28"
  Data Type Conversion1/1 -> Vout/1
  Rate Transition1/1 -> Data Type Conversion1/1
  Data Type Conversion/1 -> Rate Transition/1
  Vin/1 -> To Workspace1/1, Data Type Conversion/1
  Product3/1 -> Sum15/2
  Product1/1 -> Sum13/2
  Product4/1 -> Sum18/2
  Z25_circuit/1(Z25_out) -> Product4/2  "V25"
  Input_delay2/1 -> Z23_circuit/1(Gvar1_N), Z22_circuit/1(Gvar1_N), "LUT_Gvar1 "/1  "1"
  "LUT_Gvar1 "/1 -> Mult_delay3/1
  Product/1 -> Sum11/2
  Input_delay1/1 -> "LUT_Gvar3 "/1, Z23_circuit/3(Gvar3_N), Z24_circuit/1(Gvar3_N)  "3"
  Product2/1 -> Sum18/1
  LUT_Gvar2_rev/1 -> Mult_delay2/1
  Input_delay3/1 -> LUT_Gvar2_rev/1, Z23_circuit/2(Gvar2_N), Z25_circuit/1(Gvar2_N)  "2"
  Z24_circuit/1(Z24_out) -> Product2/2, Gain27/1  "V24"
  Sum15/1 -> Z24_circuit/2(Z24_in)  "I24"
  Delay Mod8/1 -> Z22_circuit/2(Z22_in)
  Z22_circuit/1(Z22_out) -> Product1/2, Gain30/1  "V25"
  Z23_circuit/1(Out1) -> Product5/2, Product3/2, Product/2, Gain34/1  "V24"
  Delay Mod6/1 -> Z8/1
  Sum10/1 -> Delay2/1  "I27"
  Delay2/1 -> Z27/1
  "LUT_Gvar3 "/1 -> Mult_delay1/1
  Path Delay 1/1 -> Difference3/1, To Workspace10/1, Gain5/1
  Path Delay 2/1 -> Simplify 2/1
  Path Delay 0/1 -> Simplify 1/1
  Path Delay 3/1 -> Comparator Logic/2(in_inverted)
  Path Delay 4/1 -> Sum21/2
  Delay Mod9/1 -> Z23_circuit/4(Data in)
  Mult_delay1/1 -> Product2/1, Product3/1
  Mult_delay2/1 -> Product4/1, Product5/1
  Mult_delay3/1 -> Product1/1, Product/1
  Gvar1_N/1 -> To Workspace15/1, Input_delay2/1  "1"
  Gvar2_N/1 -> To Workspace14/1, Input_delay3/1  "2"
  Product5/1 -> Z25_circuit/2(Z25_in)
  Gvar3_N/1 -> To Workspace13/1, Input_delay1/1  "3"
  Path Delay 5/1 -> Sum14/2
  Compare To Zero2/1 -> Comparator Logic/3(clk_div)
  Sum1/1 -> Switch4/1
  Input_delay4/1 -> 1-D Lookup Table1/1, To Workspace16/1  "1"
  Relational Operator4/1 -> Switch7/2
  Constant14/1 -> Switch7/1
  Gvar4_N/1 -> Input_delay4/1  "2"
  1-D Lookup Table1/1 -> Data Type Conversion2/1
  Relational Operator7/1 -> Switch4/2
  Input_delay5/1 -> Relational Operator4/2, Relational Operator7/2  "in"
  Switch4/1 -> Delay3/1
  Delay3/1 -> Switch7/3, Relational Operator4/1
  Switch7/1 -> Compare To Zero2/1, Relational Operator7/1, Sum1/2, Switch4/3  "out"
  Constant8/1 -> Sum1/1
  Data Type Conversion2/1 -> Input_delay5/1
  Gain24/1 -> Sum9/3  "I4"

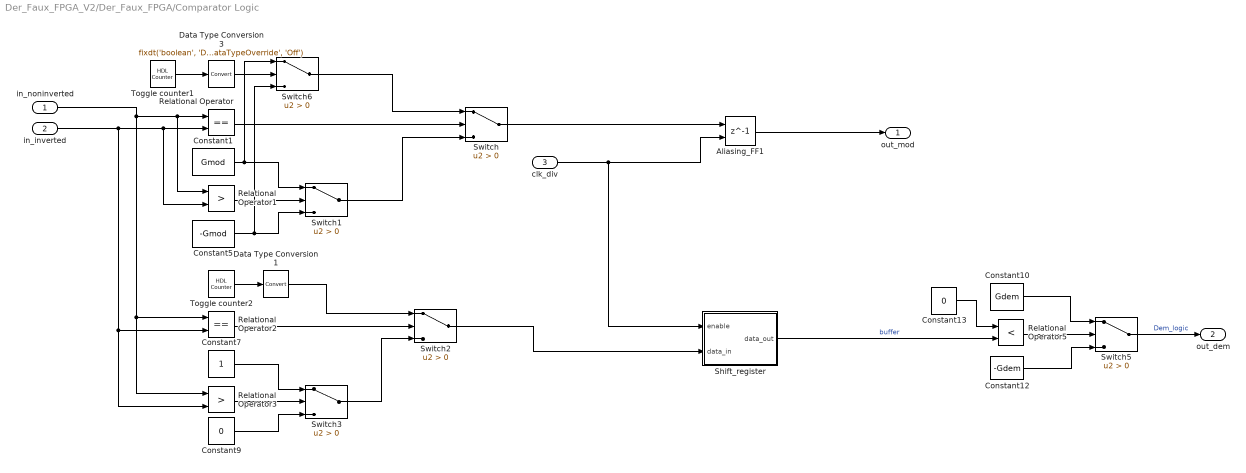
== system Der_Faux_FPGA_V2/Der_Faux_FPGA/Comparator Logic ==
  in_noninverted : Inport  OutDataTypeStr=fixdt(1,FP_len, FP_frac)  SampleTime=1/fs_sim
  in_inverted : Inport  Port=2  OutDataTypeStr=fixdt(1,FP_len, FP_frac)  SampleTime=1/fs_sim
  clk_div : Inport  Port=3  OutDataTypeStr=fixdt('boolean', 'DataTypeOverride', 'Off')  SampleTime=1/(fs_sim)  LockScale=on
  Aliasing_FF1 : Delay  DelayLength=1  InitialCondition=0  ShowEnablePort=on  SampleTime=1/(fs_sim)
      settings: InputPortMap=u0,e6
  Constant1 : Constant  Value=Gmod  OutDataTypeStr=fixdt(1,FP_len, FP_frac)  SampleTime=1/fs_sim
  Constant10 : Constant  Value=Gdem  OutDataTypeStr=fixdt(1,FP_len, FP_frac)  SampleTime=-1
  Constant12 : Constant  Value=-Gdem  OutDataTypeStr=fixdt(1,FP_len, FP_frac)  SampleTime=-1
  Constant13 : Constant  Value=0  OutDataTypeStr=fixdt('boolean', 'DataTypeOverride', 'Off')  SampleTime=1/fs_sim  LockScale=on
  Constant5 : Constant  Value=-Gmod  OutDataTypeStr=fixdt(1,FP_len, FP_frac)  SampleTime=1/fs_sim
  Constant7 : Constant  OutDataTypeStr=fixdt('boolean', 'DataTypeOverride', 'Off')  SampleTime=1/fs_sim  LockScale=on
  Constant9 : Constant  Value=0  OutDataTypeStr=fixdt('boolean', 'DataTypeOverride', 'Off')  SampleTime=1/fs_sim  LockScale=on
  Data Type Conversion1 : DataTypeConversion
  Data Type Conversion3 : DataTypeConversion  OutDataTypeStr=fixdt('boolean', 'DataTypeOverride', 'Off')  LockScale=on
  Relational Operator : RelationalOperator  Operator===  OutDataTypeStr=boolean  RndMeth=Nearest
  Relational Operator1 : RelationalOperator  Operator=>  OutDataTypeStr=boolean  RndMeth=Nearest
  Relational Operator2 : RelationalOperator  Operator===  OutDataTypeStr=fixdt('boolean', 'DataTypeOverride', 'Off')  RndMeth=Nearest
  Relational Operator3 : RelationalOperator  Operator=>  OutDataTypeStr=fixdt('boolean', 'DataTypeOverride', 'Off')  RndMeth=Nearest
  Relational Operator5 : RelationalOperator  Operator=<  OutDataTypeStr=fixdt('boolean', 'DataTypeOverride', 'Off')  RndMeth=Nearest
  Shift_register : Subsystem
  Switch{,1,5..6} (4 alike) : Switch  Criteria=u2 > Threshold  OutDataTypeStr=fixdt(1,FP_len, FP_frac)
  Switch2 : Switch  Criteria=u2 > Threshold  OutDataTypeStr=fixdt('boolean', 'DataTypeOverride', 'Off')
      settings: LockScale=on
  Switch3 : Switch  Criteria=u2 > Threshold  OutDataTypeStr=fixdt('boolean', 'DataTypeOverride', 'Off')
      settings: LockScale=on
  Toggle counter1 : hdlsllib/Sources/HDL Counter  CountType=Count limited  CountInit=0  CountStep=1  CountMax=1  CountFromType=Initial value  CountFrom=0  CountResetPort=off  CountLoadPort=off  CountEnbPort=off  CountDirPort=off  CountDataType=Unsigned  CountWordLen=1  CountFracLen=0  CountSampTime=1/fs_sim
  Toggle counter2 : hdlsllib/Sources/HDL Counter  CountType=Count limited  CountInit=0  CountStep=1  CountMax=1  CountFromType=Initial value  CountFrom=0  CountResetPort=off  CountLoadPort=off  CountEnbPort=off  CountDirPort=off  CountDataType=Unsigned  CountWordLen=1  CountFracLen=0  CountSampTime=1/fs_sim
  out_mod : Outport  OutDataTypeStr=fixdt(1,FP_len, FP_frac)  SampleTime=1/fs_sim
  out_dem : Outport  Port=2  OutDataTypeStr=fixdt(1,FP_len, FP_frac)  SampleTime=1/fs_sim
  wires:
  Constant9/1 -> Switch3/3
  Relational Operator/1 -> Switch/2
  Relational Operator1/1 -> Switch1/2
  Switch5/1 -> out_dem/1  "Dem_logic"
  in_noninverted/1 -> Relational Operator/1, Relational Operator1/1, Relational Operator3/1, Relational Operator2/1
  Constant13/1 -> Relational Operator5/1
  Relational Operator2/1 -> Switch2/2
  Switch1/1 -> Switch/3
  Relational Operator5/1 -> Switch5/2
  Constant5/1 -> Switch6/3, Switch1/3
  Constant10/1 -> Switch5/1
  Switch3/1 -> Switch2/3
  Constant1/1 -> Switch1/1, Switch6/1
  Relational Operator3/1 -> Switch3/2
  in_inverted/1 -> Relational Operator3/2, Relational Operator2/2, Relational Operator1/2, Relational Operator/2
  Constant12/1 -> Switch5/3
  Constant7/1 -> Switch3/1
  Toggle counter2/1 -> Data Type Conversion1/1
  Data Type Conversion1/1 -> Switch2/1
  Switch6/1 -> Switch/1
  Toggle counter1/1 -> Data Type Conversion3/1
  Data Type Conversion3/1 -> Switch6/2
  Switch/1 -> Aliasing_FF1/1
  clk_div/1 -> Shift_register/1(enable), Aliasing_FF1/2
  Aliasing_FF1/1 -> out_mod/1
  Shift_register/1(data_out) -> Relational Operator5/2  "buffer"
  Switch2/1 -> Shift_register/2(data_in)

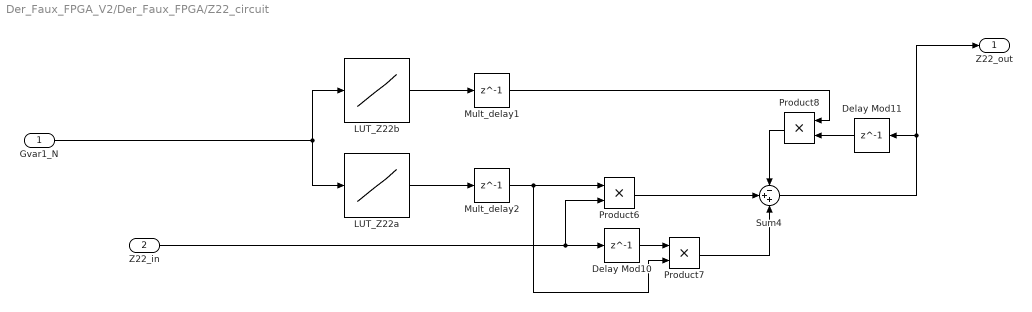
== system Der_Faux_FPGA_V2/Der_Faux_FPGA/Z22_circuit ==
  Gvar1_N : Inport  OutDataTypeStr=fixdt(0,ADC_res,0, 'DataTypeOverride', 'Off')  SampleTime=1/fs_sim  LockScale=on
  Z22_in : Inport  Port=2
  Delay Mod10 : Delay  DelayLength=1  InitialCondition=0  SampleTime=1/fs_sim
  Delay Mod11 : Delay  DelayLength=1  InitialCondition=0  SampleTime=1/fs_sim
  LUT_Z22a : Lookup_n-D  NumberOfTableDimensions=1  LookupTableObject=''  BreakpointsForDimension1=input_space  BreakpointsForDimension1FirstPoint=10  BreakpointsForDimension2FirstPoint=10  BreakpointsForDimension1Spacing=12  BreakpointsForDimension2Spacing=12  BreakpointsForDimension1DataTypeStr=Inherit: Inherit from 'Breakpoint data'  IndexSearchMethod=Evenly spaced points  Table=LUT_Z22a_opt  TableDataTypeStr=Inherit: Inherit from 'Table data'  InterpMethod=Flat  DiagnosticForOutOfRangeInput=Error  InternalRulePriority=Speed  OutDataTypeStr=Inherit: Inherit from 'Table data'  RndMeth=Simplest  InputSameDT=on  LockScale=on
  LUT_Z22b : Lookup_n-D  NumberOfTableDimensions=1  LookupTableObject=''  BreakpointsForDimension1=input_space  BreakpointsForDimension1FirstPoint=10  BreakpointsForDimension2FirstPoint=10  BreakpointsForDimension1Spacing=12  BreakpointsForDimension2Spacing=12  BreakpointsForDimension1DataTypeStr=Inherit: Inherit from 'Breakpoint data'  IndexSearchMethod=Evenly spaced points  Table=LUT_Z22b_opt  TableDataTypeStr=Inherit: Inherit from 'Table data'  InterpMethod=Flat  DiagnosticForOutOfRangeInput=Error  InternalRulePriority=Speed  OutDataTypeStr=Inherit: Inherit from 'Table data'  RndMeth=Simplest  InputSameDT=on  LockScale=on
  Mult_delay1 : Delay  DelayLength=1
  Mult_delay2 : Delay  DelayLength=1
  Product6 : Product  OutDataTypeStr=fixdt(1,FP_len, FP_frac)  SaturateOnIntegerOverflow=on
  Product7 : Product  OutDataTypeStr=fixdt(1,FP_len, FP_frac)  SaturateOnIntegerOverflow=on
  Product8 : Product  OutDataTypeStr=fixdt(1,FP_len, FP_frac)  SaturateOnIntegerOverflow=on
  Sum4 : Sum  Inputs=-++  OutDataTypeStr=fixdt(1,FP_len, FP_frac)  SaturateOnIntegerOverflow=on
  Z22_out : Outport
  wires:
  LUT_Z22b/1 -> Mult_delay1/1
  Gvar1_N/1 -> LUT_Z22b/1, LUT_Z22a/1
  Product8/1 -> Sum4/1
  Z22_in/1 -> Delay Mod10/1, Product6/2
  LUT_Z22a/1 -> Mult_delay2/1
  Product7/1 -> Sum4/3
  Delay Mod10/1 -> Product7/1
  Sum4/1 -> Z22_out/1, Delay Mod11/1
  Delay Mod11/1 -> Product8/2
  Product6/1 -> Sum4/2
  Mult_delay1/1 -> Product8/1
  Mult_delay2/1 -> Product7/2, Product6/1

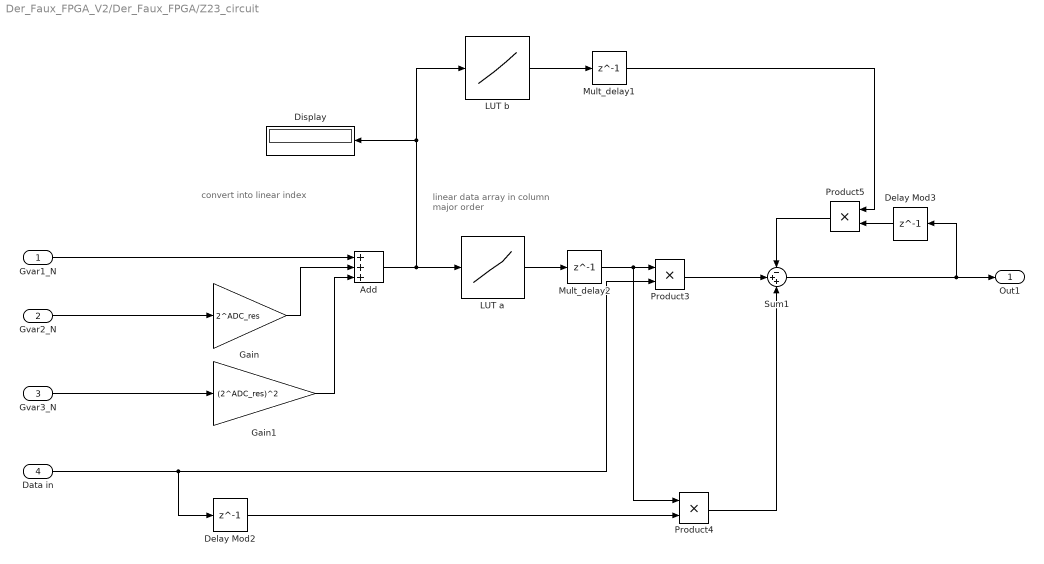
== system Der_Faux_FPGA_V2/Der_Faux_FPGA/Z23_circuit ==
  note: linear data array in
      | column major order
  note: convert into linear index
  Gvar1_N : Inport  SampleTime=1/fs_sim  LockScale=on
  Gvar2_N : Inport  Port=2  SampleTime=1/fs_sim  LockScale=on
  Gvar3_N : Inport  Port=3  SampleTime=1/fs_sim  LockScale=on
  Data in : Inport  Port=4  SampleTime=1/fs_sim  LockScale=on
  Add : Sum  Inputs=+++  AccumDataTypeStr=fixdt(0,N_ext,0)  LockScale=on
  Delay Mod2 : Delay  DelayLength=1  InitialCondition=0  SampleTime=1/fs_sim
  Delay Mod3 : Delay  DelayLength=1  InitialCondition=0  SampleTime=1/fs_sim
  Display : Display
  Gain : Gain  Gain=2^ADC_res  OutDataTypeStr=fixdt(0,N_ext,0)  LockScale=on
  Gain1 : Gain  Gain=(2^ADC_res)^2  OutDataTypeStr=fixdt(0,N_ext,0)  LockScale=on
  "LUT a " : Lookup_n-D  NumberOfTableDimensions=1  LookupTableObject=''  BreakpointsForDimension1=input_spcae_extended  BreakpointsForDimension2=0:3  BreakpointsForDimension3=0:3  BreakpointsForDimension1FirstPoint=10  BreakpointsForDimension2FirstPoint=10  BreakpointsForDimension1Spacing=12  BreakpointsForDimension2Spacing=12  BreakpointsForDimension1DataTypeStr=Inherit: Inherit from 'Breakpoint data'  BreakpointsForDimension2DataTypeStr=Inherit: Inherit from 'Breakpoint data'  BreakpointsForDimension3DataTypeStr=Inherit: Inherit from 'Breakpoint data'  IndexSearchMethod=Evenly spaced points  Table=LUT_Z23a_opt  TableDataTypeStr=Inherit: Inherit from 'Table data'  InterpMethod=Flat  DiagnosticForOutOfRangeInput=Error  InternalRulePriority=Speed  OutDataTypeStr=Inherit: Inherit from 'Table data'  RndMeth=Simplest  InputSameDT=on  LockScale=on
  LUT b : Lookup_n-D  NumberOfTableDimensions=1  LookupTableObject=''  BreakpointsForDimension1=input_spcae_extended  BreakpointsForDimension2=0:3  BreakpointsForDimension3=0:3  BreakpointsForDimension1FirstPoint=10  BreakpointsForDimension2FirstPoint=10  BreakpointsForDimension1Spacing=12  BreakpointsForDimension2Spacing=12  BreakpointsForDimension1DataTypeStr=Inherit: Inherit from 'Breakpoint data'  BreakpointsForDimension2DataTypeStr=Inherit: Inherit from 'Breakpoint data'  BreakpointsForDimension3DataTypeStr=Inherit: Inherit from 'Breakpoint data'  IndexSearchMethod=Evenly spaced points  Table=LUT_Z23b_opt  TableDataTypeStr=Inherit: Inherit from 'Table data'  InterpMethod=Flat  DiagnosticForOutOfRangeInput=Error  InternalRulePriority=Speed  OutDataTypeStr=Inherit: Inherit from 'Table data'  RndMeth=Simplest  InputSameDT=on  LockScale=on
  Mult_delay1 : Delay  DelayLength=1
  Mult_delay2 : Delay  DelayLength=1
  Product3 : Product  OutDataTypeStr=fixdt(1,FP_len, FP_frac)  SaturateOnIntegerOverflow=on
  Product4 : Product  OutDataTypeStr=fixdt(1,FP_len, FP_frac)  SaturateOnIntegerOverflow=on
  Product5 : Product  OutDataTypeStr=fixdt(1,FP_len, FP_frac)  SaturateOnIntegerOverflow=on
  Sum1 : Sum  Inputs=-++  OutDataTypeStr=fixdt(1,FP_len, FP_frac)  SaturateOnIntegerOverflow=on
  Out1 : Outport
  wires:
  Gvar2_N/1 -> Gain/1
  Gvar3_N/1 -> Gain1/1
  Gvar1_N/1 -> Add/1
  Gain/1 -> Add/2
  Gain1/1 -> Add/3
  "LUT a "/1 -> Mult_delay2/1
  Data in/1 -> Delay Mod2/1, Product3/2
  Delay Mod2/1 -> Product4/2
  Product3/1 -> Sum1/2
  Delay Mod3/1 -> Product5/2
  Product5/1 -> Sum1/1
  LUT b/1 -> Mult_delay1/1
  Sum1/1 -> Delay Mod3/1, Out1/1
  Product4/1 -> Sum1/3
  Mult_delay1/1 -> Product5/1
  Mult_delay2/1 -> Product4/1, Product3/1
  Add/1 -> Display/1, LUT b/1, "LUT a "/1

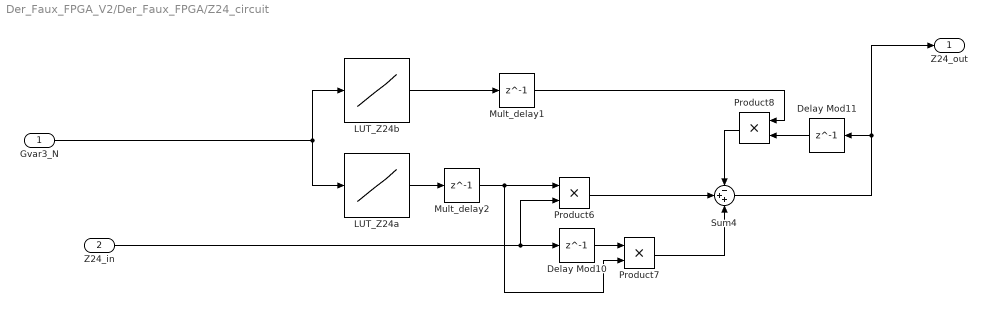
== system Der_Faux_FPGA_V2/Der_Faux_FPGA/Z24_circuit ==
  Gvar3_N : Inport  OutDataTypeStr=fixdt(0,ADC_res,0, 'DataTypeOverride', 'Off')  SampleTime=1/fs_sim  LockScale=on
  Z24_in : Inport  Port=2
  Delay Mod10 : Delay  DelayLength=1  InitialCondition=0  SampleTime=1/fs_sim
  Delay Mod11 : Delay  DelayLength=1  InitialCondition=0  SampleTime=1/fs_sim
  LUT_Z24a : Lookup_n-D  NumberOfTableDimensions=1  LookupTableObject=''  BreakpointsForDimension1=input_space  BreakpointsForDimension1FirstPoint=10  BreakpointsForDimension2FirstPoint=10  BreakpointsForDimension1Spacing=12  BreakpointsForDimension2Spacing=12  BreakpointsForDimension1DataTypeStr=Inherit: Inherit from 'Breakpoint data'  IndexSearchMethod=Evenly spaced points  Table=LUT_Z24a_opt  TableDataTypeStr=Inherit: Inherit from 'Table data'  InterpMethod=Flat  DiagnosticForOutOfRangeInput=Error  InternalRulePriority=Speed  OutDataTypeStr=Inherit: Inherit from 'Table data'  RndMeth=Simplest  InputSameDT=on  LockScale=on
  LUT_Z24b : Lookup_n-D  NumberOfTableDimensions=1  LookupTableObject=''  BreakpointsForDimension1=input_space  BreakpointsForDimension1FirstPoint=10  BreakpointsForDimension2FirstPoint=10  BreakpointsForDimension1Spacing=12  BreakpointsForDimension2Spacing=12  BreakpointsForDimension1DataTypeStr=Inherit: Inherit from 'Breakpoint data'  IndexSearchMethod=Evenly spaced points  Table=LUT_Z24b_opt  TableDataTypeStr=Inherit: Inherit from 'Table data'  InterpMethod=Flat  DiagnosticForOutOfRangeInput=Error  InternalRulePriority=Speed  OutDataTypeStr=Inherit: Inherit from 'Table data'  RndMeth=Simplest  InputSameDT=on  LockScale=on
  Mult_delay1 : Delay  DelayLength=1
  Mult_delay2 : Delay  DelayLength=1
  Product6 : Product  OutDataTypeStr=fixdt(1,FP_len, FP_frac)  SaturateOnIntegerOverflow=on
  Product7 : Product  OutDataTypeStr=fixdt(1,FP_len, FP_frac)  SaturateOnIntegerOverflow=on
  Product8 : Product  OutDataTypeStr=fixdt(1,FP_len, FP_frac)  SaturateOnIntegerOverflow=on
  Sum4 : Sum  Inputs=-++  OutDataTypeStr=fixdt(1,FP_len, FP_frac)  SaturateOnIntegerOverflow=on
  Z24_out : Outport
  wires:
  LUT_Z24b/1 -> Mult_delay1/1
  Gvar3_N/1 -> LUT_Z24b/1, LUT_Z24a/1
  Product8/1 -> Sum4/1
  Z24_in/1 -> Delay Mod10/1, Product6/2
  LUT_Z24a/1 -> Mult_delay2/1
  Product7/1 -> Sum4/3
  Delay Mod10/1 -> Product7/1
  Sum4/1 -> Z24_out/1, Delay Mod11/1
  Delay Mod11/1 -> Product8/2
  Product6/1 -> Sum4/2
  Mult_delay1/1 -> Product8/1
  Mult_delay2/1 -> Product7/2, Product6/1
